simulink model "am263px_multicore_core1"  (R2024b)
settings: Solver=FixedStepAuto  StartTime=0.0  StopTime=10.0  RelTol=1e-3
libraries: peripheral_library_blocks_am263x x2, peripheral_library_blocks_am263px x1, IPC_HWI_lib x1
settings Model: Creator=a0499511  LastModifiedBy=a0499511
settings OptimizationCC: DefaultParameterBehavior=Inlined  EnhancedBackFolding=on  PassReuseOutputArgsAs=Individual arguments  ZeroExternalMemoryAtStartup=off  ZeroInternalMemoryAtStartup=off  MaxStackSize=64  OptimizeBlockOrder=speed  DifferentSizesBufferReuse=on  OptimizationCustomize=off  EfficientTunableParamExpr=on
settings DebuggingCC: ParameterTunabilityLossMsg=error
settings HardwareCC: ProdBitPerPointer=32  ProdBitPerSizeT=32  ProdBitPerPtrDiffT=32  ProdLargestAtomicInteger=Long  ProdLargestAtomicFloat=Double  ProdWordSize=32  ProdHWDeviceType=ARM Compatible->ARM Cortex
settings SFSimCC: MATLABDynamicMemAlloc=off
settings RTWCC: Description=Embedded Coder  SystemTargetFile=ert.tlc  HardwareBoard=AM263PX LP  TemplateMakefile=ert_default_tmf  Toolchain=TI ARM Clang Compiler AM263Px | gmake
settings CodeAppCC: ForceParamTrailComments=on  IgnoreCustomStorageClasses=off  OperatorAnnotations=on  SimulinkDataObjDesc=on  SFDataObjDesc=on  InsertBlockDesc=on
settings ERTTargetCC: SupportVariableSizeSignals=on  ExtModeTransport=3  ExtModeStaticAlloc=on  ExtModeMexFile=ext_xcp  ExtModeIntrfLevel=Level2 - Open  ERTCustomFileTemplate=AM263x_codertarget_file_process.tlc

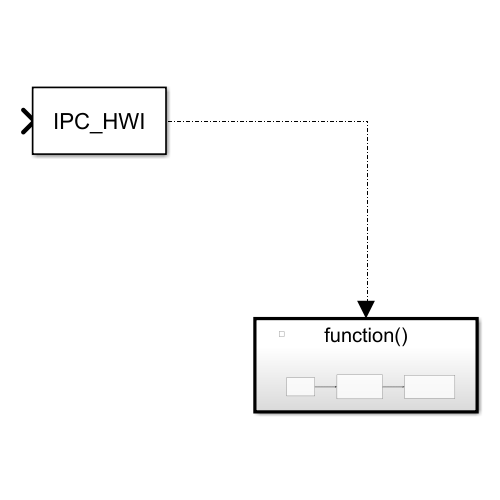
[thumbnail: Simulink's stored preview of the top-level diagram]
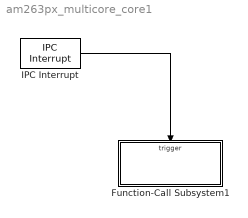
== system am263px_multicore_core1 ==
  Function-Call Subsystem1 : Subsystem  TreatAsAtomicUnit=on
  IPC Interrupt : IPC_HWI_lib/IPC Interrupt  SHOW_INPUTPORT=on
  wires:
  IPC Interrupt/1 -> Function-Call Subsystem1/Trigger

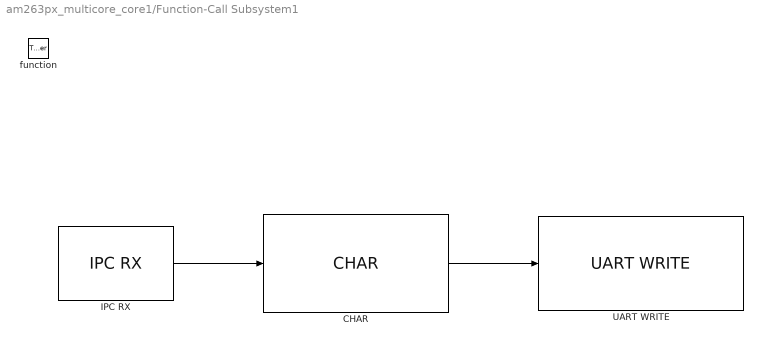
== system am263px_multicore_core1/Function-Call Subsystem1 ==
  function : TriggerPort  TriggerType=function-call  VariantControl=(inherit)
  CHAR : peripheral_library_blocks_am263x/CHAR
  IPC RX : peripheral_library_blocks_am263px/IPC RX  IPC_TXCore=R5FSS0 Core1  IPC_RXCore=R5FSS0 Core0  Input_Len=1  End_Point=13  DataType=UINT32  SampleTime=-1
  UART WRITE : peripheral_library_blocks_am263x/UART WRITE  UARTPort=UART0
  wires:
  CHAR/1 -> UART WRITE/1
  IPC RX/1 -> CHAR/1
